simulink model "person_detection"  (R2023b)
settings: Solver=FixedStepDiscrete  StartTime=0.0  StopTime=inf  FixedStep=1  RelTol=1e-3
libraries: canmsglib x2, visionsources x1
settings Model: Creator=97158  LastModifiedBy=97158
settings OptimizationCC: DefaultParameterBehavior=Inlined  EnhancedBackFolding=on  PassReuseOutputArgsAs=Individual arguments  ZeroExternalMemoryAtStartup=off  ZeroInternalMemoryAtStartup=off  OptimizeBlockOrder=speed  DifferentSizesBufferReuse=on  OptimizationCustomize=off  EfficientTunableParamExpr=on
settings DebuggingCC: ParameterTunabilityLossMsg=error
settings SFSimCC: MATLABDynamicMemAlloc=off
settings RTWCC: Description=AUTOSAR  SystemTargetFile=autosar.tlc  GenCodeOnly=on  TemplateMakefile=ert_default_tmf  DataTypeReplacement=CDataTypesFixedWidth
settings CodeAppCC: ForceParamTrailComments=on  IgnoreCustomStorageClasses=off  OperatorAnnotations=on  SimulinkDataObjDesc=on  SFDataObjDesc=on  InsertBlockDesc=on
settings STFCustomTargetCC: MultiwordLength=256  ParMdlRefBuildCompliant=on  CompOptLevelCompliant=on  IncludeMdlTerminateFcn=off  CombineOutputUpdateFcns=on  SuppressErrorStatus=on  ERTCustomFileBanners=on  SupportNonFinite=off  SupportComplex=off  SupportContinuousTime=off  SupportNonInlinedSFcns=off  RemoveResetFunc=on  MATLABClassNameForMDSCustomization=Simulink.SoftwareTarget.ERTCustomization  AutosarCompliant=on  UseToolchainInfoCompliant=on  LookupTableObjectStructAxisOrder=2,1,3,4,...  LUTObjectStructOrderEvenSpacing=Size,Table,Breakpoints  SystemTargetFile=autosar.tlc
settings ERTTargetCC: TargetLangStandard=C99 (ISO)  ConcurrentExecutionCompliant=off  IncludeMdlTerminateFcn=off  SuppressErrorStatus=on  SupportNonFinite=off  SupportComplex=off  ModelStepFunctionPrototypeControlCompliant=off  CPPClassGenCompliant=off  AutosarCompliant=on  LookupTableObjectStructAxisOrder=2,1,3,4,...  LUTObjectStructOrderEvenSpacing=Size,Table,Breakpoints  InlinedParameterPlacement=NonHierarchical  ERTCustomFileTemplate=example_file_process.tlc  BooleanTrueId=TRUE  BooleanFalseId=FALSE

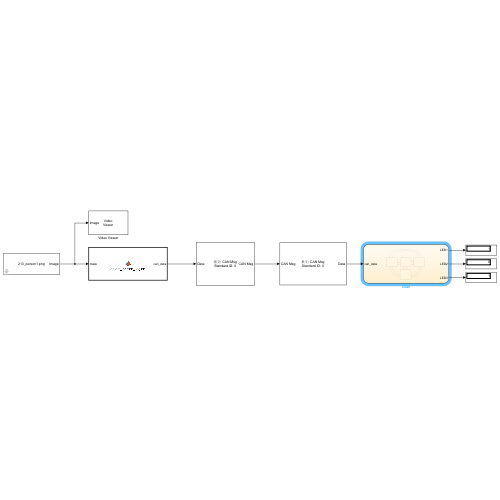
[thumbnail: Simulink's stored preview of the top-level diagram]
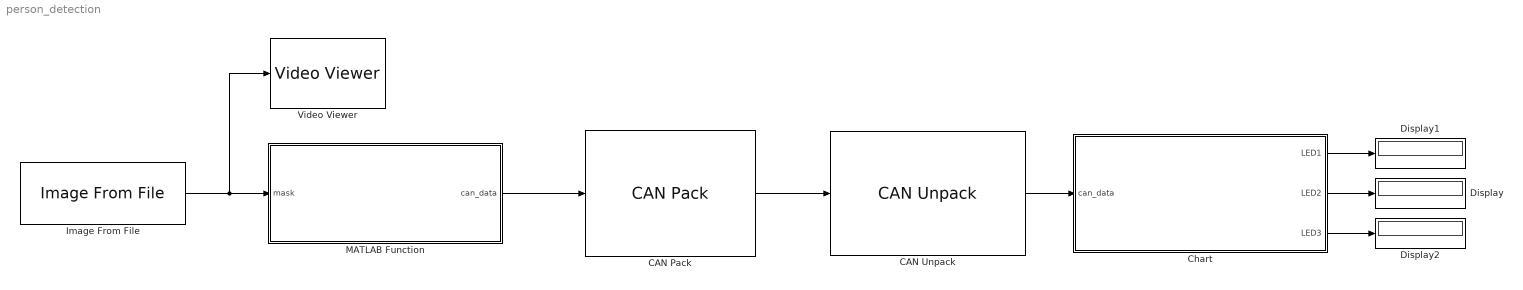
== system person_detection ==
  CAN Pack : canmsglib/CAN Pack  MsgList=(none)  MsgName=CAN Msg  MsgIDType=Standard (11-bit identifier)  MsgIdentifier=0  MsgLength=8  Remote=off  ApplyMinMax=off  BusOutput=off  SignalInfo={}
      settings: LibrarySourceBlock=canlib/CAN Pack  DataFormat=raw data
  CAN Unpack : canmsglib/CAN Unpack  MsgList=(none)  MsgName=CAN Msg  MsgIDType=Standard (11-bit identifier)  MsgIdentifier=0  MsgLength=8  SignalInfo={}  IDPort=off  TimestampPort=off  ErrorPort=off  RemotePort=off  LengthPort=off  StatusPort=off  ApplyMinMax=off
      settings: LibrarySourceBlock=canlib/CAN Unpack  DataFormat=raw data
  Chart : Stateflow chart  TreatAsAtomicUnit=on
  Display : Display
  Display1 : Display
  Display2 : Display
  Image From File : visionsources/Image From File  Tag=vipblks_nd  FileName=C:\Users\97158\Desktop\test\213_person1.png  Ts=inf  imagePorts=One multidimensional signal  OutPortLabels=R|G|B  ImageDataType=Inherit from input image  sdImageDataType=uint(8)  Signed=on  WordLength=16  FractionLengthMode=User-defined  FractionLength=15
  MATLAB Function : MATLAB Function  TreatAsAtomicUnit=on
  Video Viewer : VideoViewer  FigPos=[464.333333333333 676 418 304]
  wires:
  Image From File/1 -> Video Viewer/1, MATLAB Function/1(mask)
  MATLAB Function/1(can_data) -> CAN Pack/1
  CAN Pack/1 -> CAN Unpack/1
  CAN Unpack/1 -> Chart/1(can_data)
  Chart/2(LED2) -> Display/1
  Chart/1(LED1) -> Display1/1
  Chart/3(LED3) -> Display2/1

== matlab function person_detection/MATLAB Function ==
  data: mask input; can_data output
function can_data = detect_person_region(mask)
    % 输入：mask 为 1920x1080 的灰度图像矩阵
    width = 1920;
    region_width = width / 3;
    left_region = mask(:, 1:region_width);
    middle_region = mask(:, region_width+1:2*region_width);
    right_region = mask(:, 2*region_width+1:end);
    
    % 统计白色像素数量
    left_pixel_count = sum(left_region(:) == 255);
    middle_pixel_count = sum(middle_region(:) == 255);
    right_pixel_count = sum(right_region(:) == 255);
    
    % 找到最大区域
    pixel_counts = [left_pixel_count, middle_pixel_count, right_pixel_count];
    [max_count, max_region] = max(pixel_counts);
    
    % 生成CAN数据
    can_data = zeros(8, 1, 'uint8');
    if max_count > 0
        switch max_region
            case 1 % 左区域
                can_data(6:8) = [17; 17; 17];
            case 2 % 中间区域
                can_data(4:5) = [17; 17];
            case 3 % 右区域
                can_data(1:3) = [17; 17; 17];
        end
    end
end

== stateflow chart person_detection/Chart ==
  state Cond1
    entry:
    LED1 = false;
    LED2 = true;
    LED3 = true;
  state Default
    entry:
    LED1 = true;
    LED2 = true;
    LED3 = true;
  state Cond3
    entry:
    LED1 = true;
    LED2 = true;
    LED3 = false;
  state Cond2
    entry:
    LED1 = true;
    LED2 = false;
    LED3 = true;
  Cond3 -> Cond1 [order 1] : [can_data(1:3) == [17,17,17]]
  Cond1 -> Cond3 [order 2] : [can_data(6:8) == [17,17,17]]
  (default) -> Default
  Cond3 -> Default [order 3] : [can_data(1:8) ~= [17,17,17,17,17,17,17,17]]
  Cond1 -> Default [order 3] : [can_data(1:8) ~= [17,17,17,17,17,17,17,17,]]
  Default -> Cond1 [order 1] : [can_data(1:3) == [17,17,17]]
  Default -> Cond3 [order 3] : [can_data(6:8) == [17,17,17]]
  Cond2 -> Default [order 3] : [can_data(1:8) ~= [17,17,17,17,17,17,17,17]]
  Cond2 -> Cond1 [order 1] : [can_data(1:3) == [17,17,17]]
  Cond1 -> Cond2 [order 1] : [can_data(4:5) == [17, 17]]
  Default -> Cond2 [order 2] : [can_data(4:5) == [17,17]]
  Cond2 -> Cond3 [order 2] : [can_data(6:8) == [17,17,17]]
  Cond3 -> Cond2 [order 2] : [can_data(4:5) == [17,17]]
  data: can_data input uint8 size=8; LED1 output boolean size=1; LED2 output boolean size=1; LED3 output boolean size=1
